simulink model "sim_main_esb_5"  (R2018b)
settings: Solver=VariableStepAuto  StartTime=0.0  StopTime=10  RelTol=1e-3
values from neighbouring files (symbols this model uses):
  A_lin = subs(A_eq)    [main_sys.m]    (also in main_sys_klm.m; main_tf_10.m; main_tf_11.m; main_tf_12.m)
  B_lin = subs(B_eq)    [main_sys.m]    (also in main_sys_klm.m; main_tf_10.m; main_tf_11.m; main_tf_12.m)
  bm = 0.4e-3    (= 0.0004)    [main_cntl.m]    (also in main_sys.m = 0.00047698; main_sys_klm.m = 0.00047698; main_tf_1.m; main_tf_10.m = 0.00047698)
  C_lin = subs(C_eq)    [main_sys.m]    (also in main_sys_klm.m; main_tf_1.m = C; main_tf_10.m; main_tf_11.m)
  D_lin = zeros(1,2)    [main_sys.m]    (also in main_sys_klm.m; main_tf_10.m; main_tf_11.m; main_tf_12.m)
  dg = 0.65    [main_cntl.m]    (also in main_sys.m; main_sys_klm.m; main_tf_1.m; main_tf_10.m)
  dgs = 6    [main_cntl.m]    (also in main_sys.m; main_sys_klm.m; main_tf_1.m; main_tf_10.m)
  dh = 0.75    [main_cntl.m]    (also in main_sys.m; main_sys_klm.m; main_tf_1.m; main_tf_10.m)
  dhs = 0    [main_cntl.m]    (also in main_sys.m; main_sys_klm.m; main_tf_1.m; main_tf_10.m)
  ds = 0.001    [main_cntl.m]    (also in main_sys.m = 0; main_sys_klm.m = 0; main_tf_1.m = 0; main_tf_10.m = 0)
  J_act = [0.000306 +  0.28200e-04]    [main_cntl.m]    (also in main_sys.m; main_sys_klm.m; main_tf_1.m; main_tf_10.m)
  Jh = 5.02    [main_cntl.m]    (also in main_sys.m; main_sys_klm.m; main_tf_1.m; main_tf_10.m)
  Js_ext = 9.58e-4    (= 0.000958)    [main_cntl.m]    (also in main_sys.m; main_sys_klm.m; main_tf_1.m; main_tf_10.m)
  Js_int = 1.1e-4    (= 0.00011)    [main_cntl.m]    (also in main_sys.m; main_sys_klm.m; main_tf_1.m; main_tf_10.m)
  Kg = 2.7e4    (= 27000)    [main_cntl.m]    (also in main_sys.m; main_sys_klm.m; main_tf_1.m; main_tf_10.m)
  Kh = 1125    [main_cntl.m]    (also in main_sys.m; main_sys_klm.m; main_tf_1.m; main_tf_10.m)
  Ks = 8.1853e4*1.4    (= 114594.2)    [main_cntl.m]    (also in main_sys.m; main_sys_klm.m; main_tf_1.m; main_tf_10.m)
  rg = 160    [main_cntl.m]    (also in main_sys.m; main_sys_klm.m; main_tf_1.m; main_tf_10.m)
  Vel_mot_nom = 263    [main_cntl.m]    (also in main_sys.m; main_sys_klm.m; main_tf_1.m; main_tf_10.m)
undefined symbols (not defined in the file or in its folder): kalmf
settings Model: Creator=eshojaei  LastModifiedBy=eshojaei

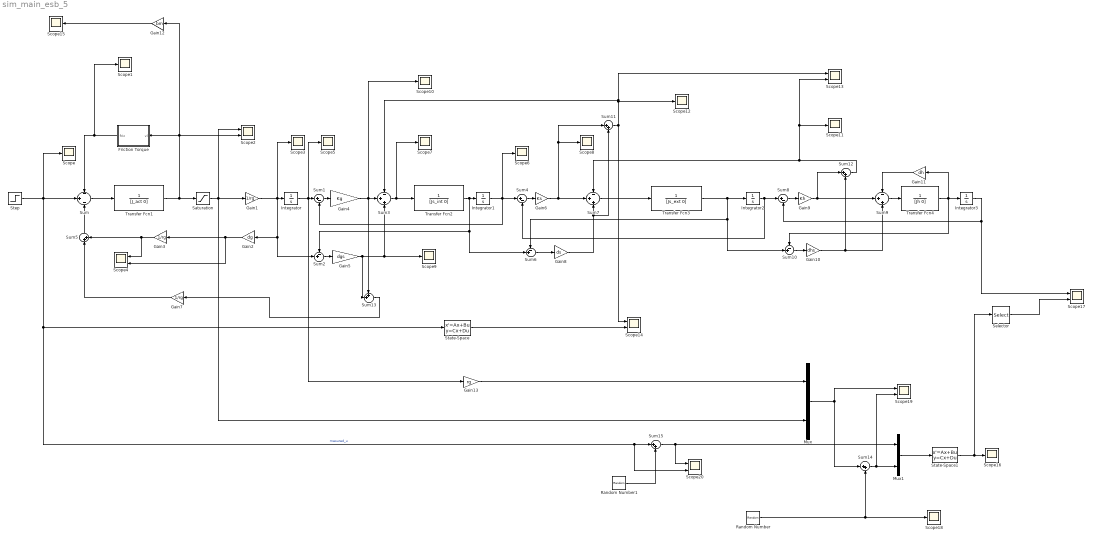
== system sim_main_esb_5 ==
  Friction Torque : MATLAB Function  TreatAsAtomicUnit=on
  Gain1 : Gain  Gain=1/rg
  Gain10 : Gain  Gain=dhs
  Gain11 : Gain  Gain=dh
  Gain12 : Gain  Gain=bm
  Gain13 : Gain  Gain=rg
  Gain2 : Gain  Gain=dg
  Gain3 : Gain  Gain=1/rg
  Gain4 : Gain  Gain=Kg
  Gain5 : Gain  Gain=dgs
  Gain6 : Gain  Gain=Ks
  Gain7 : Gain  Gain=1/rg
  Gain8 : Gain  Gain=ds
  Gain9 : Gain  Gain=Kh
  Integrator{,1..3} (4 alike) : Integrator
  Mux : Mux  Inputs=2
  Mux1 : Mux  Inputs=2
  Random Number : RandomNumber  Variance=.01  SampleTime=.001
  Random Number1 : RandomNumber  Variance=.0001  SampleTime=.001
  Saturation : Saturate  UpperLimit=Vel_mot_nom  LowerLimit=-Vel_mot_nom
  Scope{,1,3,5..12,15..16,18} (14 alike) : Scope
  Scope{2,4,13..14,17,19..20} (7 alike) : Scope  NumInputPorts=2
  Selector : Selector  InputPortWidth=10  IndexOptions=Index vector (dialog)  Indices=[9]  OutputSizes=1
  State-Space : StateSpace  A=A_lin  B=B_lin  C=C_lin  D=D_lin  InitialCondition=0
  State-Space1 : StateSpace  A=kalmf.A  B=kalmf.B  C=kalmf.C  D=kalmf.D  InitialCondition=0
  Step : Step  Time=.1  After=.04  SampleTime=0
  Sum : Sum  Inputs=-|+|-
  Sum1 : Sum  Inputs=|+-
  Sum10 : Sum  Inputs=-+|
  Sum{5,11..12,14..15} (5 alike) : Sum  Inputs=|++
  Sum13 : Sum  Inputs=++|
  Sum2 : Sum  Inputs=-+|
  Sum3 : Sum  Inputs=-++
  Sum4 : Sum  Inputs=|+-
  Sum6 : Sum  Inputs=-+|
  Sum7 : Sum  Inputs=-++
  Sum8 : Sum  Inputs=|+-
  Sum9 : Sum  Inputs=-++
  Transfer Fcn1 : TransferFcn  Denominator=[J_act 0]
  Transfer Fcn2 : TransferFcn  Denominator=[Js_int 0]
  Transfer Fcn3 : TransferFcn  Denominator=[Js_ext 0]
  Transfer Fcn4 : TransferFcn  Denominator=[Jh 0]
  wires:
  Gain6/1 -> Sum7/2, Sum11/1, Scope8/1
  Sum/1 -> Transfer Fcn1/1
  Transfer Fcn1/1 -> Saturation/1, Gain12/1, Friction Torque/1(vl), Scope2/2
  Gain4/1 -> Sum3/2, Sum13/1, Scope10/1
  Transfer Fcn2/1 -> Sum6/2, Sum2/1, Integrator1/1
  Gain7/1 -> Sum5/1
  Integrator/1 -> Gain13/1, Sum1/1, Scope5/1
  Sum1/1 -> Gain4/1
  Transfer Fcn3/1 -> Integrator2/1, Sum10/2, Sum6/1
  Sum5/1 -> Sum/3
  Sum3/1 -> Transfer Fcn2/1, Scope7/1
  Gain5/1 -> Sum3/3, Scope9/1, Sum13/2
  Gain2/1 -> Scope4/2, Gain3/1
  Gain1/1 -> Integrator/1, Scope3/1, Sum2/2, Gain2/1
  Gain3/1 -> Sum5/2, Scope4/1
  Sum2/1 -> Gain5/1
  Sum4/1 -> Gain6/1
  Sum6/1 -> Gain8/1
  Gain8/1 -> Sum11/2, Sum7/3
  Sum7/1 -> Transfer Fcn3/1
  Sum8/1 -> Gain9/1
  Gain9/1 -> Sum12/1, Sum9/2
  Sum9/1 -> Transfer Fcn4/1
  Transfer Fcn4/1 -> Gain11/1, Sum10/1, Integrator3/1
  Integrator3/1 -> Scope17/1, Sum8/2
  Gain10/1 -> Sum12/2, Sum9/3
  Sum10/1 -> Gain10/1
  Gain11/1 -> Sum9/1
  Sum11/1 -> Scope13/1, Sum3/1, Scope12/1, Scope14/1
  Sum12/1 -> Scope11/1, Scope13/2, Sum7/1
  Gain12/1 -> Scope15/1
  Sum13/1 -> Gain7/1
  Friction Torque/1(fric) -> Sum/1, Scope1/1
  State-Space/1 -> Scope14/2
  Step/1 -> Sum/2, Scope20/2, Sum15/1, State-Space/1, Scope/1  "mesured_u"
  Integrator1/1 -> Sum4/1, Scope6/1, Sum1/2
  Saturation/1 -> Mux/2, Gain1/1, Scope2/1
  Integrator2/1 -> Sum8/1, Sum4/2
  Mux1/1 -> State-Space1/1
  State-Space1/1 -> Selector/1, Scope16/1
  Gain13/1 -> Mux/1
  Random Number/1 -> Sum14/2, Scope18/1
  Sum14/1 -> Scope19/2, Mux1/2
  Mux/1 -> Sum14/1, Scope19/1
  Sum15/1 -> Scope20/1, Mux1/1
  Random Number1/1 -> Sum15/2
  Selector/1 -> Scope17/2

== matlab function sim_main_esb_5/Friction Torque ==
  data: vl input; fric output
function fric = fcn(vl)

    
   fric = (5981672325465929*vl)/147573952589676412928 + (7059617857129123*tanh((6072588977179245*vl)/36028797018963968))/144115188075855872 + (2558104915892175*tanh((5176012883402097*vl)/576460752303423488))/72057594037927936;
